simulink model "SIM"  (R2024b)
settings: Solver=VariableStepAuto  StartTime=0.0  StopTime=TF  FixedStep=0.1  MaxStep=0.1  RelTol=1e-3
values from neighbouring files (symbols this model uses):
  x0 = [38 ... (first row only)    [Initilise_Constants.m]    (also in test.m = [85)
  z0 = -500    [Initilise_Constants.m]
undefined symbols (not defined in the file or in its folder): CntrlDeflec, control, etatoTrim, toNormalAxis, UAV_model3
settings Model: Creator=Will  LastModifiedBy=Will

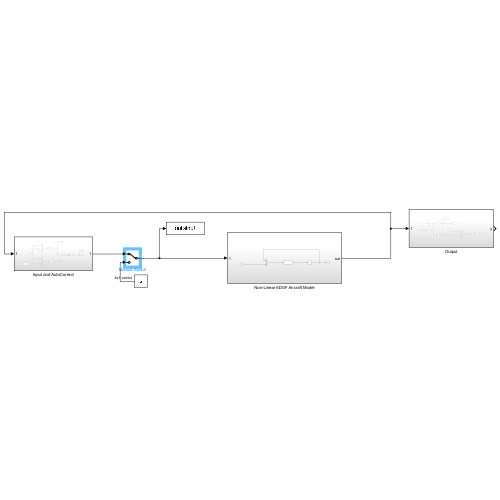
[thumbnail: Simulink's stored preview of the top-level diagram]
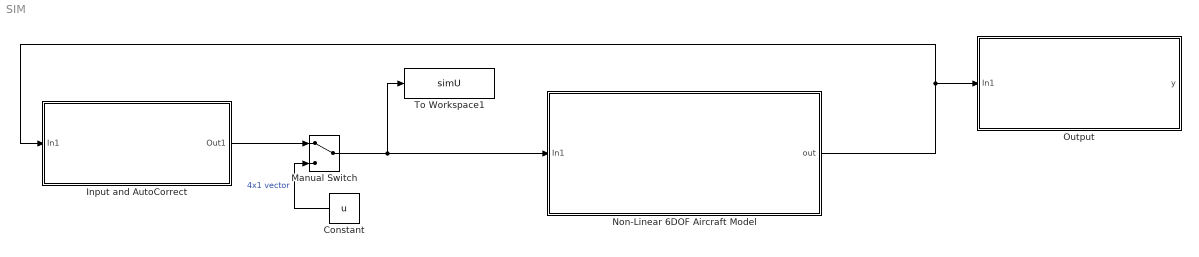
== system SIM ==
  Constant : Constant  Value=u
  Input and AutoCorrect : Subsystem
  Manual Switch : ManualSwitch
  Non-Linear 6DOF Aircraft Model : Subsystem
  Output : Subsystem
  To Workspace1 : ToWorkspace  VariableName=simU  SaveFormat=Timeseries  SampleTime=-1
  wires:
  Non-Linear 6DOF Aircraft Model/1(out) -> Input and AutoCorrect/1(In1), Output/1(In1)
  Constant/1 -> Manual Switch/2  "4x1 vector"
  Input and AutoCorrect/1(Out1) -> Manual Switch/1
  Manual Switch/1 -> Non-Linear 6DOF Aircraft Model/1(In1), To Workspace1/1

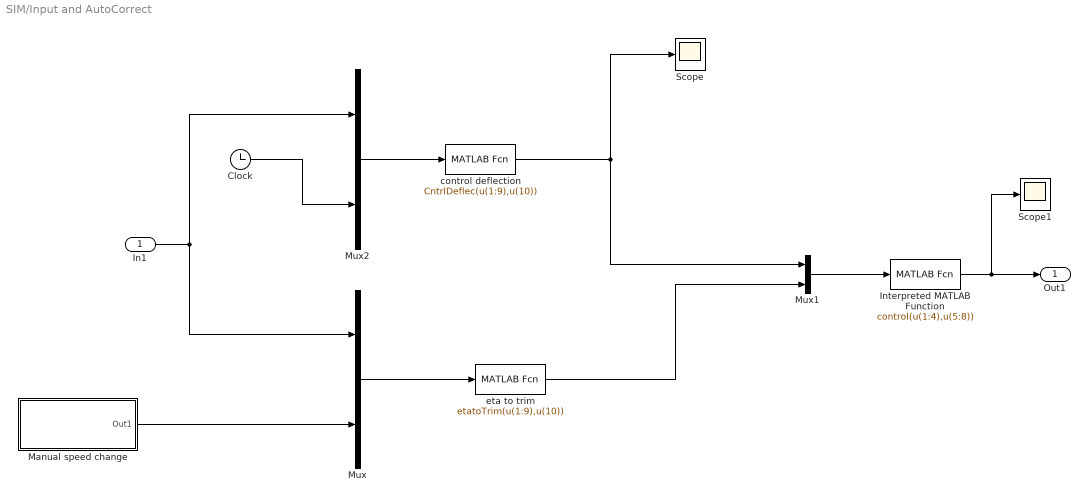
== system SIM/Input and AutoCorrect ==
  In1 : Inport
  Clock : Clock
  Interpreted MATLAB Function : MATLABFcn  MATLABFcn=control(u(1:4),u(5:8))
  Manual speed change : Subsystem
  Mux : Mux  Inputs=2
  Mux1 : Mux  Inputs=2
  Mux2 : Mux  Inputs=2
  Scope : Scope
  Scope1 : Scope
  control deflection : MATLABFcn  MATLABFcn=CntrlDeflec(u(1:9),u(10))
  eta to trim : MATLABFcn  MATLABFcn=etatoTrim(u(1:9),u(10))
  Out1 : Outport
  wires:
  In1/1 -> Mux2/1, Mux/1
  Mux/1 -> eta to trim/1
  Manual speed change/1(Out1) -> Mux/2
  Clock/1 -> Mux2/2
  Mux2/1 -> control deflection/1
  control deflection/1 -> Scope/1, Mux1/1
  eta to trim/1 -> Mux1/2
  Mux1/1 -> Interpreted MATLAB Function/1
  Interpreted MATLAB Function/1 -> Scope1/1, Out1/1

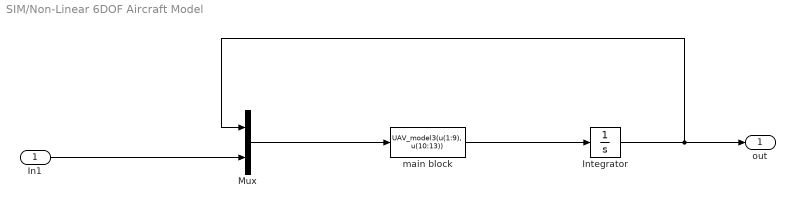
== system SIM/Non-Linear 6DOF Aircraft Model ==
  In1 : Inport
  Integrator : Integrator  InitialCondition=x0
  Mux : Mux  Inputs=2
  main block : MATLABFcn  MATLABFcn=UAV_model3(u(1:9), u(10:13))
  out : Outport
  wires:
  Integrator/1 -> out/1, Mux/1
  In1/1 -> Mux/2
  Mux/1 -> main block/1
  main block/1 -> Integrator/1

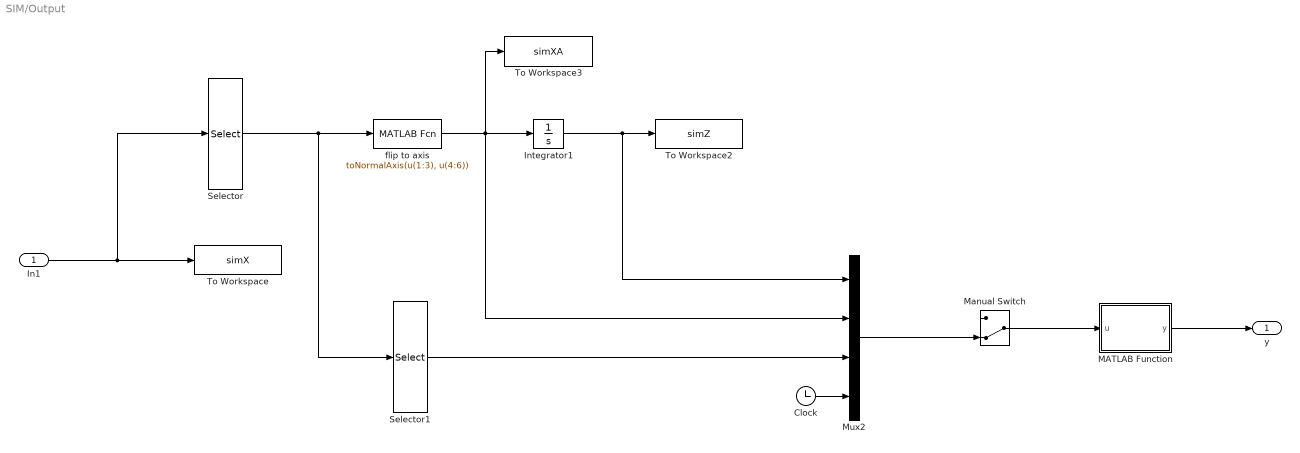
== system SIM/Output ==
  In1 : Inport
  Clock : Clock
  Integrator1 : Integrator  InitialCondition=z0
  MATLAB Function : MATLAB Function  TreatAsAtomicUnit=on
  Manual Switch : ManualSwitch  CurrentSetting=0
  Mux2 : Mux
  Selector : Selector  InputPortWidth=9  IndexOptions=Index vector (dialog)  Indices=[1 2 3 7 8 9]  OutputSizes=1
  Selector1 : Selector  InputPortWidth=6  IndexOptions=Index vector (dialog)  Indices=[4 5 6]  OutputSizes=1
  To Workspace : ToWorkspace  VariableName=simX  SaveFormat=Timeseries  SampleTime=-1
  To Workspace2 : ToWorkspace  VariableName=simZ  SaveFormat=Timeseries  SampleTime=-1
  To Workspace3 : ToWorkspace  VariableName=simXA  SaveFormat=Timeseries  SampleTime=-1
  flip to axis : MATLABFcn  MATLABFcn=toNormalAxis(u(1:3), u(4:6))
  y : Outport
  wires:
  Integrator1/1 -> To Workspace2/1, Mux2/1
  Selector/1 -> flip to axis/1, Selector1/1
  In1/1 -> To Workspace/1, Selector/1
  flip to axis/1 -> To Workspace3/1, Integrator1/1, Mux2/2
  Selector1/1 -> Mux2/3
  MATLAB Function/1(y) -> y/1
  Clock/1 -> Mux2/4
  Mux2/1 -> Manual Switch/2
  Manual Switch/1 -> MATLAB Function/1(u)

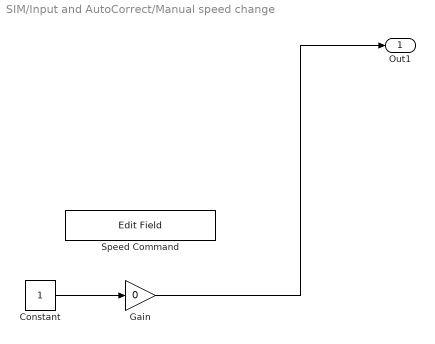
== system SIM/Input and AutoCorrect/Manual speed change ==
  Constant : Constant
  Gain : Gain  Gain=0
  Speed Command : EditField  LabelPosition=Hide  ShowInitialText=on  Alignment=Center
  Out1 : Outport
  wires:
  Constant/1 -> Gain/1
  Gain/1 -> Out1/1

== matlab function SIM/Output/MATLAB Function ==
  data: u input; y output
function y = fcn(u)
coder.extrinsic('real_time_plot');
real_time_plot(u);
y = u;
